simulink library "model_lib"  (Simulink 6.3)
undefined symbols (not defined in the file or in its folder): ADQUANT, alt_alp, alt_delt, alt_gamma, alt_ht, alt_R, alt_T0, atmos, att_trim_IC, constants, dc_L2W_IC, DiscIntNeverNeededParam, dtsim, enforce_fuel, inertia_maxprop, inertia_noprop, latlonh_IC, MACH, MACH_att_int_IC, MACH_att_Kb, MACH_att_Kc, MACH_att_Ki, MACH_pos_IC, MACH_pos_int_IC, MACH_pos_Kb, MACH_pos_Kc, MACH_pos_Ki, MACH_pqr_IC, MACH_pqr_int_IC, MACH_pqr_Kb, MACH_pqr_Kc, MACH_pqr_Ki, MACH_quat_IC, MACH_vel_IC, MACH_vel_int_IC, MACH_vel_Kb, MACH_vel_Kc, MACH_vel_Ki, mass_maxprop, mass_noprop, obac_params, r_accel, r_cg_maxprop, r_cg_noprop, r_prop, rho_sl, SENS, SERVO, throttle_idx, tvc_idx, use_NdEdh_pos, use_wind_meas_sim, use_xdot_ground, vehicle_params
libraries: utility_lib x22, model_lib x18, simulink x14, aerospace x1
(part 1 of 2)
settings Model: LastModifiedBy=E700252  ExtModeAutoUpdateStatusClock=off  StrictBusMsg=None

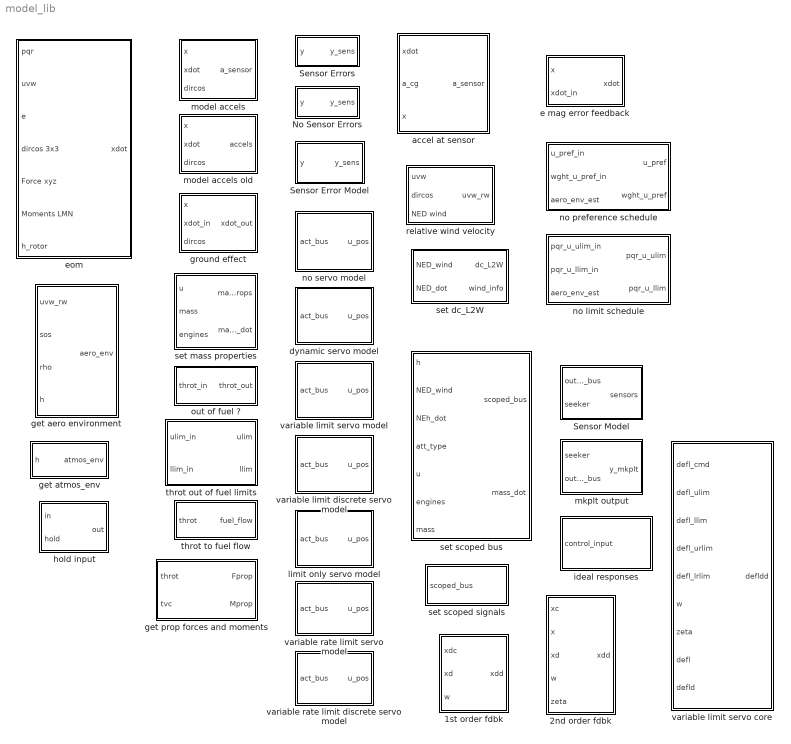
== system model_lib ==
  1st order fdbk : Subsystem
  2nd order fdbk : Subsystem
  No Sensor Errors : Subsystem
  Sensor Error Model : Subsystem  BlockChoice=No Sensor Errors
      settings: TemplateBlock=self  MemberBlocks=No Sensor Errors,Sensor Errors
  Sensor Errors : Subsystem
  Sensor Model : Subsystem
  accel at sensor : Subsystem  mask{vehicle_params=vehicle_params}
      mask prompts: vehicle_params "vehicle params"
      mask init:
      | paramnames = fieldnames(vehicle_params);
      | for i=1:length(paramnames)
      | 	eval([paramnames{i} '= vehicle_params.' paramnames{i} ';']);
      | end
  dynamic servo model : Subsystem
  e mag error feedback : Subsystem
  eom : Subsystem
  get aero environment : Subsystem
  get atmos_env : Subsystem  mask{atmos_params=atmos}
      mask prompts: atmos_params "atmos params"
      mask init:
      | paramnames = fieldnames(atmos_params);
      | for i=1:length(paramnames)
      | 	eval([paramnames{i} '= atmos_params.' paramnames{i} ';']);
      | end
  get prop forces and moments : Subsystem
  ground effect : Subsystem  mask{vehicle_params=vehicle_params}
      mask prompts: vehicle_params "vehicle params"
      mask init:
      | num_x = vehicle_params.num_x;
  hold input : Subsystem
  ideal responses : Subsystem
  limit only servo model : Subsystem
  mkplt output : Subsystem
  model accels : Subsystem  mask{vehicle_params=vehicle_params}
      mask prompts: vehicle_params "vehicle params"
      mask init:
      | paramnames = fieldnames(vehicle_params);
      | for i=1:length(paramnames)
      | 	eval([paramnames{i} '= vehicle_params.' paramnames{i} ';']);
      | end
  model accels old : Subsystem  mask{vehicle_params=vehicle_params}
      mask prompts: vehicle_params "vehicle params"
      mask init:
      | lxa = vehicle_params.lxa;
      | lya = vehicle_params.lya;
      | lza = vehicle_params.lza;
      | num_x = vehicle_params.num_x;
      | 
      | if isfield(vehicle_params,'zero_pqr_dot')
      | 	zero_pqr_dot = vehicle_params.zero_pqr_dot;
      | else
      | 	zero_pqr_dot = 0;
      | end
  no limit schedule : Subsystem
  no preference schedule : Subsystem
  no servo model : Subsystem
  out of fuel ? : Subsystem
  relative wind velocity : Subsystem
  set dc_L2W : Subsystem
  set mass properties : Subsystem  mask{vehicle_params=vehicle_params}
      mask prompts: vehicle_params "vehicle params"
      mask init:
      | paramnames = fieldnames(vehicle_params);
      | for i=1:length(paramnames)
      | 	eval([paramnames{i} '= vehicle_params.' paramnames{i} ';']);
      | end
  set scoped bus : Subsystem  mask{vehicle_params=obac_params}
      mask prompts: vehicle_params "vehicle params"
  set scoped signals : Subsystem
  throt out of fuel limits : Subsystem
  throt to fuel flow : Subsystem
  variable limit discrete servo model : Subsystem
  variable limit servo core : Subsystem
  variable limit servo model : Subsystem
  variable rate limit discrete servo model : Subsystem
  variable rate limit servo model : Subsystem

== system model_lib/1st order fdbk ==
  xdc : Inport
  xd : Inport  Port=2
  w : Inport  Port=3
  Product1 : Product  RndMeth=Zero
  Sum1 : Sum  Inputs=|+-
  xdd : Outport
  wires:
  Product1/1 -> xdd/1
  w/1 -> Product1/2
  xd/1 -> Sum1/2
  xdc/1 -> Sum1/1
  Sum1/1 -> Product1/1

== system model_lib/2nd order fdbk ==
  xc : Inport
  x : Inport  Port=2
  xd : Inport  Port=3
  w : Inport  Port=4
  zeta : Inport  Port=5
  Gain : Gain  Gain=2
  Product1 : Product  Inputs=3  RndMeth=Zero
  Product2 : Product  Inputs=3  RndMeth=Zero
  Sum1 : Sum  Inputs=|+-
  Sum2 : Sum  Inputs=|+-
  xdd : Outport
  wires:
  Gain/1 -> Product2/2
  xd/1 -> Product2/3
  zeta/1 -> Gain/1
  Product2/1 -> Sum2/2
  Sum2/1 -> xdd/1
  Product1/1 -> Sum2/1
  w/1 -> Product2/1, Product1/3, Product1/2
  x/1 -> Sum1/2
  xc/1 -> Sum1/1
  Sum1/1 -> Product1/1

== system model_lib/No Sensor Errors ==
  note: Sensors
  y : Inport
  y_sens : Outport
  wires:
  y/1 -> y_sens/1

== system model_lib/Sensor Error Model ==
  y : Inport
  No Sensor Errors : model_lib/No Sensor Errors
  y_sens : Outport
  wires:
  y/1 -> No Sensor Errors/1
  No Sensor Errors/1 -> y_sens/1

== system model_lib/Sensor Errors ==
  note: Sensors
  y : Inport
  Sensor A/D Quantization : Subsystem
  Sensor Errors : Subsystem
  y_sens : Outport
  wires:
  Sensor Errors/1(ys) -> Sensor A/D Quantization/1(y)
  Sensor A/D Quantization/1(yQ) -> y_sens/1
  y/1 -> Sensor Errors/1(y)

== system model_lib/Sensor Model ==
  note: Note: dircos is the DCM
      | for the quaternion state
  output_bus : Inport
  seeker : Inport  Port=2
  Bus Creator : BusCreator  Inputs=9
  Bus Selector : BusSelector  OutputSignals=x,xdot,y.accels_cg,y.dircos,u_servo,NED_wind
  Constant : Constant
  Gain1 : Gain  Gain=[1 1 -1]  SaturateOnIntegerOverflow=on
  NEh : Selector  Elements=MACH.NEh_idx  InputPortWidth=MACH.num_x
  NEh2LLh : utility_lib/NEh2LLh
  NEh_dot : Selector  Elements=MACH.NEh_idx  InputPortWidth=MACH.num_x
  Signal Specification : SignalSpecification
  Terminator : Terminator
  initial position : Constant  Value=latlonh_IC
  pqr : Selector  Elements=MACH.pqr_idx  InputPortWidth=MACH.num_x
  quat : Selector  Elements=MACH.quat_idx  InputPortWidth=MACH.num_x
  use_wind_meas_sim : Gain  Gain=use_wind_meas_sim  SaturateOnIntegerOverflow=on
  sensors : Outport
  wires:
  Bus Selector/4 -> Terminator/1  "<dircos>"
  Bus Selector/3 -> Bus Creator/5  "<accels_cg>"
  Bus Selector/1 -> pqr/1, NEh/1, quat/1  "<x>"
  seeker/1 -> Bus Creator/9  "seeker"
  Bus Selector/6 -> use_wind_meas_sim/1  "<NED_wind>"
  output_bus/1 -> Bus Selector/1
  NEh/1 -> NEh2LLh/1
  Constant/1 -> Bus Creator/6  "nav_ok"
  initial position/1 -> NEh2LLh/2
  quat/1 -> Bus Creator/3  "e"
  Bus Selector/2 -> NEh_dot/1  "<xdot>"
  NEh_dot/1 -> Gain1/1  "NEh_dot"
  Bus Creator/1 -> sensors/1
  pqr/1 -> Bus Creator/1  "pqr"
  NEh2LLh/1 -> Bus Creator/2  "latlonh"
  Gain1/1 -> Bus Creator/4  "NED_dot"
  use_wind_meas_sim/1 -> Bus Creator/8  "NED_wind"
  Bus Selector/5 -> Signal Specification/1  "<u_servo>"
  Signal Specification/1 -> Bus Creator/7  "u_meas"

== system model_lib/accel at sensor ==
  xdot : Inport
  a_cg : Inport  Port=2
  x : Inport  Port=3
  Product : Product  RndMeth=Zero
  Product1 : Product  RndMeth=Zero
  Sum : Sum  Inputs=+-|
  Sum1 : Sum  Inputs=|+-  SaturateOnIntegerOverflow=on  InputSameDT=on
  Sum10 : Sum  Inputs=+++  SaturateOnIntegerOverflow=on  InputSameDT=on
  accel location : Constant  Value=r_accel
  pqr : Selector  Elements=pqr_idx  InputPortWidth=num_x
  pqr . l_sensor : simulink/Math Operations/Dot Product  InputSameDT=on  OutDataType=sfix(16)  OutScaling=2^-10  DoSatur=off
  pqr . pqr : simulink/Math Operations/Dot Product  InputSameDT=on  OutDataType=sfix(16)  OutScaling=2^-10  DoSatur=off
  pqr_dot : Selector  Elements=pqr_idx  InputPortWidth=num_x
  pqr_dot x l_sensor : utility_lib/cross product
  a_sensor : Outport
  wires:
  Sum1/1 -> Sum10/3
  pqr_dot x l_sensor/1 -> Sum10/2
  a_cg/1 -> Sum10/1
  Product1/1 -> Sum1/2
  Product/1 -> Sum1/1
  pqr . pqr/1 -> Product1/2
  pqr . l_sensor/1 -> Product/1
  x/1 -> pqr/1
  xdot/1 -> pqr_dot/1
  Sum10/1 -> a_sensor/1
  accel location/1 -> Sum/1
  [r_cg] -> Sum/2
  Sum/1 -> Product1/1, pqr . l_sensor/1, pqr_dot x l_sensor/2  "l_sensor"
  pqr_dot/1 -> pqr_dot x l_sensor/1
  pqr/1 -> Product/2, pqr . pqr/2, pqr . pqr/1, pqr . l_sensor/2

== system model_lib/dynamic servo model ==
  note: DYNAMIC SERVO MODEL
      | W^2*e^(-sT) / (S^2 + 2*Z*Ws + W^2)
  act_bus : Inport
  2*Z*W : Gain  Orientation=left  Gain=2*SERVO.z.*SERVO.w  SaturateOnIntegerOverflow=on
  Bus Selector : BusSelector  OutputSignals=u_cmd
  Sum : Sum  Inputs=|+-  SaturateOnIntegerOverflow=on  InputSameDT=on
  Sum1 : Sum  Inputs=|+-  SaturateOnIntegerOverflow=on  InputSameDT=on
  Transport Delay : TransportDelay  DelayTime=SERVO.delay  InitialOutput=SERVO.x0  PadeOrder=2
  W^2 : Gain  Gain=SERVO.w.^2  SaturateOnIntegerOverflow=on
  pos integrator : Integrator  InitialCondition=SERVO.x0  LimitOutput=on  UpperSaturationLimit=SERVO.ulim  LowerSaturationLimit=SERVO.llim
  rate integrator : Integrator  LimitOutput=on  UpperSaturationLimit=SERVO.urlim  LowerSaturationLimit=SERVO.lrlim
  u_pos : Outport
  wires:
  Sum/1 -> W^2/1
  W^2/1 -> Sum1/1
  2*Z*W/1 -> Sum1/2
  rate integrator/1 -> 2*Z*W/1, pos integrator/1
  pos integrator/1 -> Sum/2, u_pos/1
  Sum1/1 -> rate integrator/1
  act_bus/1 -> Bus Selector/1
  Transport Delay/1 -> Sum/1
  Bus Selector/1 -> Transport Delay/1  "<u_cmd>"

== system model_lib/e mag error feedback ==
  x : Inport
  xdot_in : Inport  Port=2
  Assignment : Assignment  Elements=MACH.quat_idx  OutputInitialize=Initialize using input (U1)
  Constant : Constant  Orientation=up
  Constant2 : Constant  Value=0.001
  Gain : Gain  Gain=MACH.K_quaterr/2  SaturateOnIntegerOverflow=on
  Math Function1 : Math  Operator=reciprocal  SaturateOnIntegerOverflow=on
  Math Function2 : Math  Operator=square  SaturateOnIntegerOverflow=on
  MinMax : MinMax  Function=max  Inputs=2
  Product2 : Product  Inputs=**  SaturateOnIntegerOverflow=on  InputSameDT=on
  Sum1 : Sum  Inputs=|-+  SaturateOnIntegerOverflow=on  InputSameDT=on
  Sum2 : Sum  Inputs=+  SaturateOnIntegerOverflow=on  InputSameDT=on
  Sum3 : Sum  Inputs=|++  SaturateOnIntegerOverflow=on  InputSameDT=on
  quat : Selector  Elements=MACH.quat_idx  InputPortWidth=MACH.num_x
  quatdot : Selector  Elements=MACH.quat_idx  InputPortWidth=MACH.num_x
  xdot : Outport
  wires:
  Gain/1 -> Product2/2
  Sum1/1 -> Gain/1
  Constant/1 -> Sum1/2
  Math Function1/1 -> Sum1/1
  Math Function2/1 -> Sum2/1
  Constant2/1 -> MinMax/2
  Sum2/1 -> MinMax/1
  MinMax/1 -> Math Function1/1
  x/1 -> quat/1
  xdot_in/1 -> quatdot/1, Assignment/1
  quat/1 -> Product2/1, Math Function2/1
  Sum3/1 -> Assignment/2
  quatdot/1 -> Sum3/1
  Product2/1 -> Sum3/2
  Assignment/1 -> xdot/1

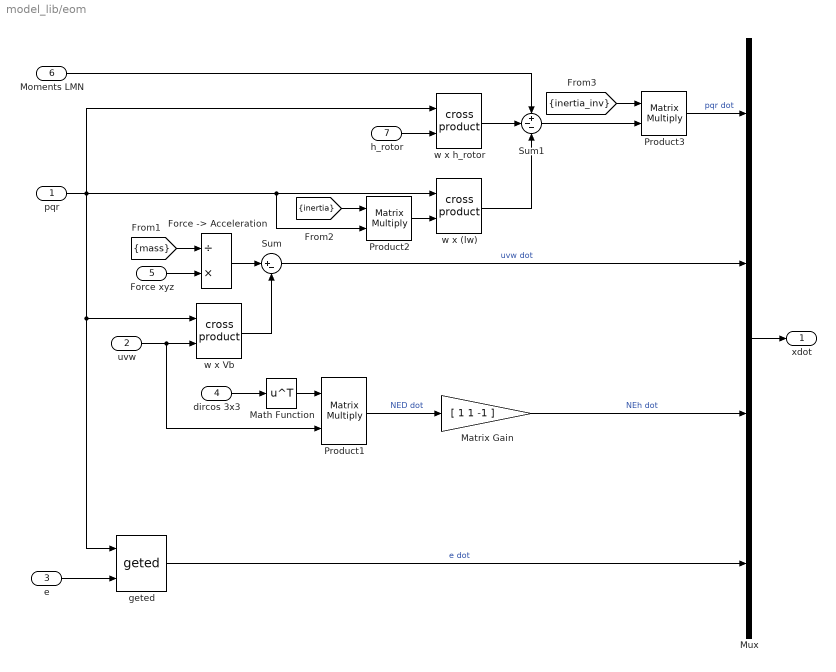
== system model_lib/eom ==
  pqr : Inport
  uvw : Inport  Port=2
  e : Inport  Port=3
  dircos 3x3 : Inport  Port=4
  "Force xyz " : Inport  Port=5
  Moments LMN : Inport  Port=6
  h_rotor : Inport  Port=7
  "Force -> Acceleration" : Product  Inputs=/*  RndMeth=Zero
  Math Function : Math  Operator=transpose  SaturateOnIntegerOverflow=on
  Matrix Gain : Gain  Gain=[ 1 1 -1 ]  SaturateOnIntegerOverflow=on
  Mux : Mux
  Product1 : Product  Multiplication=Matrix(*)  SaturateOnIntegerOverflow=on  InputSameDT=on
  Product2 : Product  Multiplication=Matrix(*)  RndMeth=Zero
  Product3 : Product  Multiplication=Matrix(*)  RndMeth=Zero
  Sum : Sum  Inputs=|+-  SaturateOnIntegerOverflow=on
  Sum1 : Sum  Inputs=+--  SaturateOnIntegerOverflow=on
  geted : utility_lib/geted
  w x (lw) : utility_lib/cross product
  w x Vb : utility_lib/cross product
  w x h_rotor : utility_lib/cross product
  xdot : Outport
  wires:
  Mux/1 -> xdot/1
  geted/1 -> Mux/4  "e dot"
  e/1 -> geted/2
  uvw/1 -> Product1/2, w x Vb/2
  w x Vb/1 -> Sum/2
  "Force xyz "/1 -> "Force -> Acceleration"/2
  Sum/1 -> Mux/2  "uvw dot"
  Matrix Gain/1 -> Mux/3  "NEh dot"
  dircos 3x3/1 -> Math Function/1
  pqr/1 -> geted/1, w x Vb/1, Product2/2, w x (lw)/1, w x h_rotor/1
  Product3/1 -> Mux/1  "pqr dot"
  Product2/1 -> w x (lw)/2
  Moments LMN/1 -> Sum1/1
  Sum1/1 -> Product3/2
  Product1/1 -> Matrix Gain/1  "NED dot"
  Math Function/1 -> Product1/1
  "Force -> Acceleration"/1 -> Sum/1
  h_rotor/1 -> w x h_rotor/2
  w x (lw)/1 -> Sum1/3
  w x h_rotor/1 -> Sum1/2
  [inertia] -> Product2/1
  [mass] -> "Force -> Acceleration"/1
  [inertia_inv] -> Product3/1

== system model_lib/get aero environment ==
  uvw_rw : Inport
  sos : Inport  Port=2  PortDimensions=1
  rho : Inport  Port=3  PortDimensions=1
  h : Inport  Port=4  PortDimensions=1
  Bus Creator : BusCreator  Inputs=9
  Constant : Constant  Value=0.0001
  MinMax : MinMax  Function=max  Inputs=2
  Product1 : Product  RndMeth=Zero
  Product2 : Product  Inputs=*/  RndMeth=Zero
  Signal Specification : SignalSpecification  Dimensions=1
  uvw_rw2Vab : utility_lib/uvw_rw2Vab
  wind_qbar : Fcn  Expr=0.5*u^2
  aero_env : Outport
  wires:
  uvw_rw/1 -> Bus Creator/9, uvw_rw2Vab/1  "uvw_rw"
  uvw_rw2Vab/1 -> MinMax/2
  h/1 -> Bus Creator/8  "h"
  Constant/1 -> MinMax/1
  MinMax/1 -> wind_qbar/1, Product2/1, Signal Specification/1
  Product1/1 -> Bus Creator/4  "qbar"
  rho/1 -> Product1/1, Bus Creator/3  "rho"
  wind_qbar/1 -> Product1/2
  uvw_rw2Vab/3 -> Bus Creator/7  "beta"
  sos/1 -> Product2/2, Bus Creator/2  "sos"
  Product2/1 -> Bus Creator/1  "Mach"
  Bus Creator/1 -> aero_env/1
  Signal Specification/1 -> Bus Creator/5  "vel"
  uvw_rw2Vab/2 -> Bus Creator/6  "alpha"

== system model_lib/get atmos_env ==
  h : Inport
  Bus Creator : BusCreator  Inputs=5
  Gain : Gain  Gain=alt_R*constants.g
  Gain1 : Gain  Gain=alt_gamma*alt_R*constants.g
  Math Function : Math  Operator=sqrt  SaturateOnIntegerOverflow=on
  Product : Product  RndMeth=Zero
  air density : Subsystem
  air temp : Subsystem
  atmos_env : Outport
  wires:
  h/1 -> air temp/1(h), Bus Creator/5, air density/1(h)  "h"
  air temp/1(T) -> Gain1/1, Bus Creator/3, Product/2  "T"
  Gain1/1 -> Math Function/1
  Math Function/1 -> Bus Creator/4  "sos"
  Bus Creator/1 -> atmos_env/1
  air density/1(rho) -> Bus Creator/1, Product/1  "rho"
  Product/1 -> Gain/1
  Gain/1 -> Bus Creator/2  "P"

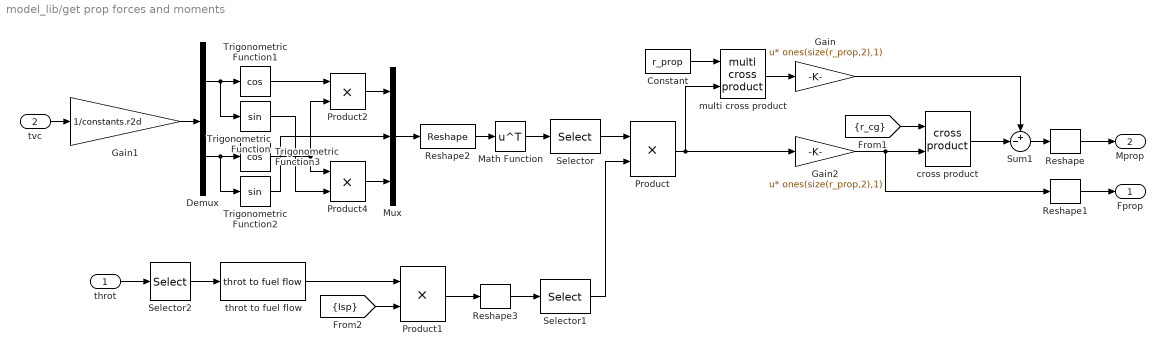
== system model_lib/get prop forces and moments ==
  throt : Inport
  tvc : Inport  Port=2
  Constant : Constant  Value=r_prop  VectorParams1D=off
  Demux : Demux  Outputs=2
  Gain : Gain  Gain=ones(size(r_prop,2),1)  Multiplication=Matrix(u*K)
  Gain1 : Gain  Gain=1/constants.r2d
  Gain2 : Gain  Gain=ones(size(r_prop,2),1)  Multiplication=Matrix(u*K)
  Math Function : Math  Operator=transpose  SaturateOnIntegerOverflow=on
  Mux : Mux  Inputs=3
  Product{,1..2,4} (4 alike) : Product  RndMeth=Zero
  Reshape : simulink/Math Operations/Reshape  OutputDimensionality=1-D array  OutputDimensions=[1,1]
  Reshape1 : simulink/Math Operations/Reshape  OutputDimensionality=1-D array  OutputDimensions=[1,1]
  Reshape2 : simulink/Math Operations/Reshape  OutputDimensionality=Customize  OutputDimensions=[length(tvc_idx)/2 3]
  Reshape3 : simulink/Math Operations/Reshape  OutputDimensionality=Row vector  OutputDimensions=[1,1]
  Selector : Selector  InputType=Matrix  Elements=[1 3]  Rows=-1  Columns=tvc_select  InputPortWidth=3
  Selector1 : Selector  InputType=Matrix  Elements=[1 3]  Rows=ones(1,size(r_prop,2))  Columns=-1  InputPortWidth=3
  Selector2 : Selector  Elements=throt_select  InputPortWidth=length(throttle_idx)
  Sum1 : Sum  Inputs=+-|
  Trigonometric Function : Trigonometry
  Trigonometric Function1 : Trigonometry  Operator=cos
  Trigonometric Function2 : Trigonometry
  Trigonometric Function3 : Trigonometry  Operator=cos
  cross product : utility_lib/cross product
  multi cross product : utility_lib/multi cross product
  throt to fuel flow : model_lib/throt to fuel flow
  Fprop : Outport
  Mprop : Outport  Port=2
  wires:
  Reshape3/1 -> Selector1/1
  Selector1/1 -> Product/2
  Selector/1 -> Product/1
  Math Function/1 -> Selector/1
  Reshape2/1 -> Math Function/1
  Reshape1/1 -> Fprop/1
  Reshape/1 -> Mprop/1
  Sum1/1 -> Reshape/1
  cross product/1 -> Sum1/2
  Gain/1 -> Sum1/1
  multi cross product/1 -> Gain/1
  Gain2/1 -> cross product/2, Reshape1/1
  [r_cg] -> cross product/1
  Product/1 -> multi cross product/2, Gain2/1
  Constant/1 -> multi cross product/1
  tvc/1 -> Gain1/1
  Demux/1 -> Trigonometric Function1/1, Trigonometric Function/1
  Demux/2 -> Trigonometric Function3/1, Trigonometric Function2/1
  Product4/1 -> Mux/3
  Trigonometric Function3/1 -> Product2/2, Product4/1
  throt/1 -> Selector2/1
  Gain1/1 -> Demux/1
  Product2/1 -> Mux/1
  Trigonometric Function1/1 -> Product2/1
  Trigonometric Function/1 -> Product4/2
  Trigonometric Function2/1 -> Mux/2
  [Isp] -> Product1/2
  throt to fuel flow/1 -> Product1/1
  Mux/1 -> Reshape2/1
  Product1/1 -> Reshape3/1
  Selector2/1 -> throt to fuel flow/1

== system model_lib/ground effect ==
  x : Inport
  xdot_in : Inport  Port=2
  dircos : Inport  Port=3
  Matrix Gain1 : Gain  Gain=use_xdot_ground  SaturateOnIntegerOverflow=on
  Selector2 : Selector  Elements=MACH.NEh_idx(3)  InputPortWidth=num_x
  above ground ? : Switch  Criteria=u2 > Threshold  SaturateOnIntegerOverflow=on
  include ground effect : Subsystem
  xdot_out : Outport
  wires:
  xdot_in/1 -> include ground effect/1(xdot_in), above ground ?/1
  dircos/1 -> include ground effect/3(dircos)
  above ground ?/1 -> xdot_out/1
  Selector2/1 -> above ground ?/2  "h"
  x/1 -> include ground effect/2(x), Selector2/1
  Matrix Gain1/1 -> above ground ?/3
  include ground effect/1(xdot_out) -> Matrix Gain1/1

== system model_lib/hold input ==
  in : Inport
  hold : Inport  Port=2
  Constant : Constant
  Memory : Memory  InheritSampleTime=on
  Memory1 : Memory  Orientation=left  InheritSampleTime=on
  Product : Product  RndMeth=Zero
  Switch : Switch  Criteria=u2 ~= 0
  out : Outport
  wires:
  hold/1 -> Product/1
  in/1 -> Switch/3
  Constant/1 -> Memory/1
  Memory/1 -> Product/2
  Product/1 -> Switch/2
  Switch/1 -> out/1, Memory1/1
  Memory1/1 -> Switch/1

== system model_lib/ideal responses ==
  control_input : Inport
      settings: BusObject=control_input_bus
  ideal att rate response : Subsystem
  ideal pos vel response : Subsystem
  wires:
  control_input/1 -> ideal pos vel response/1(control_input), ideal att rate response/1(control_input)

== system model_lib/limit only servo model ==
  note: LIMIT ONLY SERVO MODEL
  act_bus : Inport
  Bus Selector1 : BusSelector  OutputSignals=effector_limits.u_ulim,effector_limits.u_llim,u_cmd
  Enforce lower limit : MinMax  Function=max  Inputs=2  OutScaling=2^-10  ZeroCross=off
  Enforce upper limit : MinMax  Inputs=2  OutScaling=2^-10  ZeroCross=off
  Rate Limiter : RateLimiter  RisingSlewLimit=SERVO.urlim  FallingSlewLimit=SERVO.lrlim  SampleTimeMode=inherited  InitialCondition=SERVO.x0
  u_pos : Outport
  wires:
  Rate Limiter/1 -> u_pos/1
  Enforce lower limit/1 -> Enforce upper limit/2
  Bus Selector1/1 -> Enforce upper limit/1  "<u_ulim>"
  Enforce upper limit/1 -> Rate Limiter/1
  act_bus/1 -> Bus Selector1/1
  Bus Selector1/3 -> Enforce lower limit/2  "<u_cmd>"
  Bus Selector1/2 -> Enforce lower limit/1  "<u_llim>"

== system model_lib/mkplt output ==
  seeker : Inport
  output_bus : Inport  Port=2
  Bus Creator1 : BusCreator  Inputs=10
  Bus Selector : BusSelector  OutputSignals=y.dircos,x,NED_wind
  Bus Selector1 : BusSelector  OutputSignals=mass_props.mass,atmos_env.P,atmos_env.T,dc_L2W
  Gain : Gain  SaturateOnIntegerOverflow=on
  angles : Subsystem
  order outputs as expected by mkplt : BusSelector  OutputSignals=output_bus.y.accels,output_bus.y.accels_cg,output_bus.y.dircos,uvw_rw,tilta;tiltb;cam,phi;theta;psi,mu;alpha;beta,mass,output_bus.y.aero_env,P,T,seeker  OutputAsBus=on
  uvw : Selector  Elements=MACH.uvw_idx  InputPortWidth=MACH.num_x
  y_mkplt : Outport
  wires:
  Bus Selector1/4 -> Bus Creator1/10  "<dc_L2W>"
  Bus Selector1/3 -> Bus Creator1/9  "<T>"
  Bus Selector1/2 -> Bus Creator1/8  "<P>"
  Bus Selector1/1 -> Bus Creator1/7  "<mass>"
  seeker/1 -> Bus Creator1/6  "seeker"
  [scoped_bus] -> Bus Selector1/1
  Bus Selector/2 -> uvw/1  "<x>"
  Bus Creator1/1 -> order outputs as expected by mkplt/1
  Bus Selector/3 -> angles/3(NED_wind)  "<NED_wind>"
  uvw/1 -> angles/2(uvw)
  Bus Selector/1 -> angles/1(dircos)  "<dircos>"
  Gain/1 -> y_mkplt/1
  order outputs as expected by mkplt/1 -> Gain/1
  output_bus/1 -> Bus Creator1/1, Bus Selector/1  "output_bus"
  angles/3(phi;theta;psi) -> Bus Creator1/4  "phi;theta;psi"
  angles/2(tilta;tiltb;cam) -> Bus Creator1/3  "tilta;tiltb;cam"
  angles/1(uvw_rw) -> Bus Creator1/2  "uvw_rw"
  angles/4(mu;alpha;beta) -> Bus Creator1/5  "mu;alpha;beta"

== system model_lib/model accels ==
  x : Inport
  xdot : Inport  Port=2
  dircos : Inport  Port=3
  Gain2 : Gain  Gain=constants.g  SaturateOnIntegerOverflow=on
  accel at cg : Subsystem
  accel at sensor : model_lib/accel at sensor  vehicle_params=vehicle_params
  dircos(:,3) : Selector  Elements=7:9  InputPortWidth=9
  pqr : Selector  Elements=pqr_idx  InputPortWidth=num_x
  uvw : Selector  Elements=uvw_idx  InputPortWidth=num_x
  uvw_dot : Selector  Elements=uvw_idx  InputPortWidth=num_x
  a_sensor : Outport
  wires:
  x/1 -> uvw/1, pqr/1, accel at sensor/3
  dircos(:,3)/1 -> Gain2/1
  xdot/1 -> uvw_dot/1, accel at sensor/1
  dircos/1 -> dircos(:,3)/1
  uvw_dot/1 -> accel at cg/1(uvw_dot)
  accel at sensor/1 -> a_sensor/1
  accel at cg/1(a_cg) -> accel at sensor/2
  Gain2/1 -> accel at cg/2(gvec)
  uvw/1 -> accel at cg/3(uvw)
  pqr/1 -> accel at cg/4(pqr)

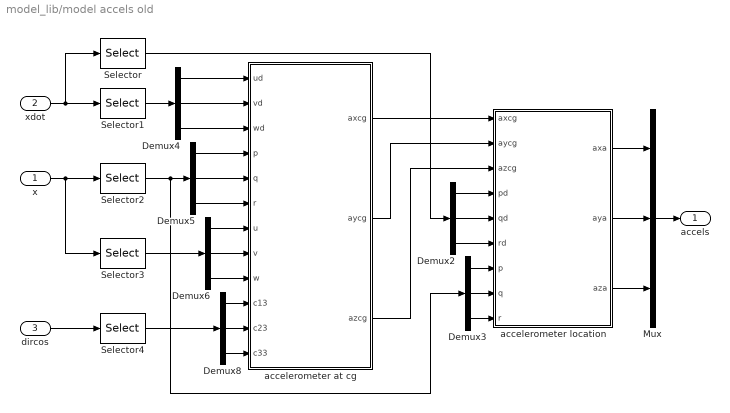
== system model_lib/model accels old ==
  x : Inport
  xdot : Inport  Port=2
  dircos : Inport  Port=3
  Demux{2..6,8} (6 alike) : Demux  Outputs=3
  Mux : Mux  Inputs=[1 1 1]
  Selector : Selector  Elements=MACH.pqr_idx  InputPortWidth=num_x
  Selector1 : Selector  Elements=MACH.uvw_idx  InputPortWidth=num_x
  Selector2 : Selector  Elements=MACH.pqr_idx  InputPortWidth=num_x
  Selector3 : Selector  Elements=MACH.uvw_idx  InputPortWidth=num_x
  Selector4 : Selector  Elements=7:9  InputPortWidth=9
  accelerometer at cg : Subsystem
  accelerometer location : Subsystem
  accels : Outport
  wires:
  accelerometer at cg/1(axcg) -> accelerometer location/1(axcg)
  accelerometer at cg/2(aycg) -> accelerometer location/2(aycg)
  accelerometer at cg/3(azcg) -> accelerometer location/3(azcg)
  Mux/1 -> accels/1
  accelerometer location/1(axa) -> Mux/1
  accelerometer location/2(aya) -> Mux/2
  accelerometer location/3(aza) -> Mux/3
  Demux2/1 -> accelerometer location/4(pd)
  Demux2/2 -> accelerometer location/5(qd)
  Demux2/3 -> accelerometer location/6(rd)
  Demux3/1 -> accelerometer location/7(p)
  Demux3/2 -> accelerometer location/8(q)
  Demux3/3 -> accelerometer location/9(r)
  Demux4/1 -> accelerometer at cg/1(ud)
  Demux4/2 -> accelerometer at cg/2(vd)
  Demux5/1 -> accelerometer at cg/4(p)
  Demux5/2 -> accelerometer at cg/5(q)
  Demux5/3 -> accelerometer at cg/6(r)
  Demux6/1 -> accelerometer at cg/7(u)
  Demux6/2 -> accelerometer at cg/8(v)
  Demux6/3 -> accelerometer at cg/9(w)
  Demux4/3 -> accelerometer at cg/3(wd)
  Selector1/1 -> Demux4/1
  Selector2/1 -> Demux5/1, Demux3/1
  Selector3/1 -> Demux6/1
  dircos/1 -> Selector4/1
  Demux8/1 -> accelerometer at cg/10(c13)
  Demux8/2 -> accelerometer at cg/11(c23)
  Demux8/3 -> accelerometer at cg/12(c33)
  xdot/1 -> Selector1/1, Selector/1
  Selector4/1 -> Demux8/1
  x/1 -> Selector2/1, Selector3/1
  Selector/1 -> Demux2/1

== system model_lib/no limit schedule ==
  note: NO LIMIT SCHEDULE
  pqr_u_ulim_in : Inport
  pqr_u_llim_in : Inport  Port=2
  aero_env_est : Inport  Port=3
  Terminator : Terminator
  pqr_u_ulim : Outport
  pqr_u_llim : Outport  Port=2
  wires:
  pqr_u_llim_in/1 -> pqr_u_llim/1
  pqr_u_ulim_in/1 -> pqr_u_ulim/1
  aero_env_est/1 -> Terminator/1

== system model_lib/no preference schedule ==
  note: NO PREFERENCE SCHEDULE
  u_pref_in : Inport
  wght_u_pref_in : Inport  Port=2
  aero_env_est : Inport  Port=3
  Terminator : Terminator
  u_pref : Outport
  wght_u_pref : Outport  Port=2
  wires:
  u_pref_in/1 -> u_pref/1
  wght_u_pref_in/1 -> wght_u_pref/1
  aero_env_est/1 -> Terminator/1

== system model_lib/no servo model ==
  note: NO SERVO MODEL
  act_bus : Inport
  Bus Selector : BusSelector  OutputSignals=u_cmd
  u_pos : Outport
  wires:
  act_bus/1 -> Bus Selector/1
  Bus Selector/1 -> u_pos/1  "<u_cmd>"

== system model_lib/out of fuel ? ==
  throt_in : Inport
  Compare To Zero : simulink/Logic and Bit Operations/Compare To Zero  relop=<=  LogicOutDataTypeMode=boolean  ZeroCross=off
  Constant : Constant  Value=enforce_fuel
  Logical Operator : Logic  Operator=NAND  AllPortsSameDT=off  OutDataTypeMode=Boolean
  Product : Product  RndMeth=Zero
  throt_out : Outport
  wires:
  Product/1 -> throt_out/1
  [fuel] -> Compare To Zero/1
  throt_in/1 -> Product/1
  Compare To Zero/1 -> Logical Operator/1
  Constant/1 -> Logical Operator/2
  Logical Operator/1 -> Product/2

== system model_lib/relative wind velocity ==
  uvw : Inport
  dircos : Inport  Port=2
  NED wind : Inport  Port=3
  Product : Product  Multiplication=Matrix(*)  SaturateOnIntegerOverflow=on
  Reshape : simulink/Math Operations/Reshape  OutputDimensionality=Customize  OutputDimensions=[3,3]
  Sum1 : Sum  Inputs=++|  SaturateOnIntegerOverflow=on
  uvw_rw : Outport
  wires:
  dircos/1 -> Reshape/1
  uvw/1 -> Sum1/2
  NED wind/1 -> Product/2
  Product/1 -> Sum1/1
  Sum1/1 -> uvw_rw/1
  Reshape/1 -> Product/1

== system model_lib/set dc_L2W ==
  NED_wind : Inport
  NED_dot : Inport  Port=2
  Bus Creator : BusCreator  Inputs=3
  Bus Selector : BusSelector  OutputSignals=Rslant,azimuth,elevation
  Signal Specification : SignalSpecification
  Signal Specification1 : SignalSpecification
  Signal Specification2 : SignalSpecification
  Sum : Sum  Inputs=|++
  vec2dc : utility_lib/vec2dc
  dc_L2W : Outport
  wind_info : Outport  Port=2
  wires:
  Sum/1 -> vec2dc/1
  NED_wind/1 -> Sum/1
  NED_dot/1 -> Sum/2
  vec2dc/1 -> dc_L2W/1
  vec2dc/2 -> Bus Selector/1
  Bus Selector/1 -> Signal Specification/1  "<Rslant>"
  Bus Selector/2 -> Signal Specification1/1  "<azimuth>"
  Bus Selector/3 -> Signal Specification2/1  "<elevation>"
  Bus Creator/1 -> wind_info/1
  Signal Specification/1 -> Bus Creator/1  "vel_rw"
  Signal Specification1/1 -> Bus Creator/2  "chi_rw"
  Signal Specification2/1 -> Bus Creator/3  "gamma_rw"

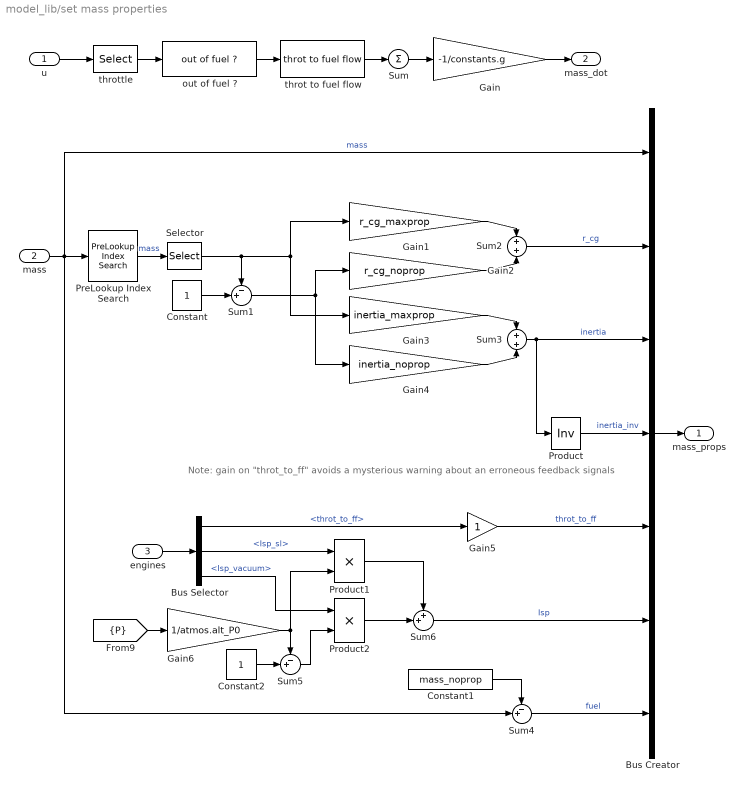
== system model_lib/set mass properties ==
  note: Note: gain on "throt_to_ff" avoids
      |  a mysterious warning about an
      | erroneous feedback signals
  u : Inport
  mass : Inport  Port=2
  engines : Inport  Port=3
  Bus Creator : BusCreator  Inputs=7
  Bus Selector : BusSelector  OutputSignals=throt_to_ff,Isp_sl,Isp_vacuum
  Constant : Constant
  Constant1 : Constant  Value=mass_noprop
  Constant2 : Constant
  Gain : Gain  Gain=-1/constants.g
  Gain1 : Gain  Gain=r_cg_maxprop
  Gain2 : Gain  Gain=r_cg_noprop
  Gain3 : Gain  Gain=inertia_maxprop
  Gain4 : Gain  Gain=inertia_noprop
  Gain5 : Gain
  Gain6 : Gain  Gain=1/atmos.alt_P0
  PreLookup Index Search : simulink/Lookup Tables/PreLookup Index Search  bpData=[mass_noprop max(mass_maxprop,mass_noprop+1)]  searchMode=Binary Search  cacheBpFlag=off  outputFlag=off  IndexDataType=uint32  extrapMode=Clip to Range  rangeErrorMode=None
  Product : Product  Inputs=/  Multiplication=Matrix(*)  RndMeth=Zero
  Product1 : Product  RndMeth=Zero
  Product2 : Product  RndMeth=Zero
  Selector : Selector  Elements=2  InputPortWidth=2
  Sum : Sum  Inputs=+
  Sum1 : Sum  Inputs=-+|
  Sum2 : Sum  Inputs=+|+
  Sum3 : Sum  Inputs=+|+
  Sum4 : Sum  Inputs=-+|
  Sum5 : Sum  Inputs=-+|
  Sum6 : Sum  Inputs=++|
  out of fuel ? : model_lib/out of fuel ?
  throt to fuel flow : model_lib/throt to fuel flow
  throttle : Selector  Elements=MACH.throttle_idx  InputPortWidth=MACH.num_u
  mass_props : Outport
  mass_dot : Outport  Port=2
  wires:
  Gain5/1 -> Bus Creator/5  "throt_to_ff"
  Product2/1 -> Sum6/2
  Product1/1 -> Sum6/1
  Sum5/1 -> Product2/2
  Constant2/1 -> Sum5/2
  Gain6/1 -> Sum5/1, Product1/2
  Bus Selector/3 -> Product2/1  "<Isp_vacuum>"
  [P] -> Gain6/1
  Bus Selector/2 -> Product1/1  "<Isp_sl>"
  engines/1 -> Bus Selector/1
  Product/1 -> Bus Creator/4  "inertia_inv"
  Constant1/1 -> Sum4/1
  Sum4/1 -> Bus Creator/7  "fuel"
  out of fuel ?/1 -> throt to fuel flow/1
  Gain/1 -> mass_dot/1
  Sum3/1 -> Bus Creator/3, Product/1  "inertia"
  Sum2/1 -> Bus Creator/2  "r_cg"
  Gain4/1 -> Sum3/2
  Gain3/1 -> Sum3/1
  Gain2/1 -> Sum2/2
  Gain1/1 -> Sum2/1
  Sum1/1 -> Gain4/1, Gain2/1
  Constant/1 -> Sum1/2
  Selector/1 -> Gain3/1, Gain1/1, Sum1/1
  mass/1 -> Bus Creator/1, Sum4/2, PreLookup Index Search/1  "mass"
  Sum/1 -> Gain/1
  throt to fuel flow/1 -> Sum/1
  Bus Creator/1 -> mass_props/1
  throttle/1 -> out of fuel ?/1
  u/1 -> throttle/1
  Sum6/1 -> Bus Creator/6  "Isp"
  PreLookup Index Search/1 -> Selector/1  "mass"
  Bus Selector/1 -> Gain5/1  "<throt_to_ff>"

== system model_lib/set scoped bus ==
  note: Note: gain on "att_type" avoids
      |  a mysterious warning about an
      | erroneous feedback signals
  h : Inport
  NED_wind : Inport  Port=2
  NEh_dot : Inport  Port=3
  att_type : Inport  Port=4
  u : Inport  Port=5
  engines : Inport  Port=6
  mass : Inport  Port=7
  Bus Creator : BusCreator  Inputs=5
  Gain : Gain  Gain=[1 1 -1]  SaturateOnIntegerOverflow=on
  Gain1 : Gain
  get atmos_env : model_lib/get atmos_env  atmos_params=atmos
  set dc_L2W : model_lib/set dc_L2W
  set mass properties : model_lib/set mass properties  vehicle_params=vehicle_params
  scoped_bus : Outport
  mass_dot : Outport  Port=2
  wires:
  Gain1/1 -> Bus Creator/4  "att_type"
  engines/1 -> set mass properties/3
  Gain/1 -> set dc_L2W/2
  mass/1 -> set mass properties/2
  att_type/1 -> Gain1/1
  NEh_dot/1 -> Gain/1
  h/1 -> get atmos_env/1
  u/1 -> set mass properties/1
  NED_wind/1 -> set dc_L2W/1
  set dc_L2W/1 -> Bus Creator/2  "dc_L2W"
  Bus Creator/1 -> scoped_bus/1
  set mass properties/2 -> mass_dot/1
  set mass properties/1 -> Bus Creator/5  "mass_props"
  get atmos_env/1 -> Bus Creator/1  "atmos_env"
  set dc_L2W/2 -> Bus Creator/3  "wind_info"

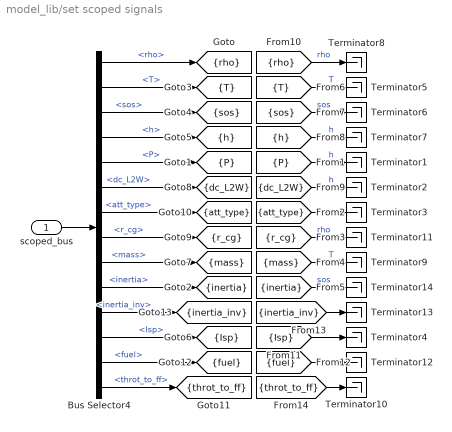
== system model_lib/set scoped signals ==
  scoped_bus : Inport
  Bus Selector4 : BusSelector  OutputSignals=atmos_env.rho,atmos_env.T,atmos_env.sos,atmos_env.h,atmos_env.P,dc_L2W,att_type,mass_props.r_cg,mass_props.mass,mass_props.inertia,mass_props.inertia_inv,mass_props.Isp,mass_props.fuel,mass_props.throt_to_ff
  Terminator{1..14} (14 alike) : Terminator
  tag scope: Isp=scoped, P=scoped, T=scoped, att_type=scoped, dc_L2W=scoped, fuel=scoped, h=scoped, inertia=scoped, inertia_inv=scoped, mass=scoped, r_cg=scoped, rho=scoped, sos=scoped, throt_to_ff=scoped
  wires:
  [throt_to_ff] -> Terminator10/1
  Bus Selector4/14 -> [throt_to_ff]  "<throt_to_ff>"
  Bus Selector4/11 -> [inertia_inv]  "<inertia_inv>"
  [inertia_inv] -> Terminator13/1
  [fuel] -> Terminator12/1
  Bus Selector4/13 -> [fuel]  "<fuel>"
  [Isp] -> Terminator4/1
  [inertia] -> Terminator14/1  "sos"
  [mass] -> Terminator9/1  "T"
  [r_cg] -> Terminator11/1  "rho"
  [att_type] -> Terminator3/1
  [dc_L2W] -> Terminator2/1  "h"
  [P] -> Terminator1/1  "h"
  [rho] -> Terminator8/1  "rho"
  [T] -> Terminator5/1  "T"
  [sos] -> Terminator6/1  "sos"
  [h] -> Terminator7/1  "h"
  Bus Selector4/12 -> [Isp]  "<Isp>"
  Bus Selector4/10 -> [inertia]  "<inertia>"
  Bus Selector4/9 -> [mass]  "<mass>"
  Bus Selector4/8 -> [r_cg]  "<r_cg>"
  Bus Selector4/7 -> [att_type]  "<att_type>"
  Bus Selector4/6 -> [dc_L2W]  "<dc_L2W>"
  Bus Selector4/5 -> [P]  "<P>"
  Bus Selector4/4 -> [h]  "<h>"
  Bus Selector4/3 -> [sos]  "<sos>"
  Bus Selector4/2 -> [T]  "<T>"
  Bus Selector4/1 -> [rho]  "<rho>"
  scoped_bus/1 -> Bus Selector4/1

== system model_lib/throt out of fuel limits ==
  ulim_in : Inport
  llim_in : Inport  Port=2
  Assignment : Assignment  Elements=MACH.throttle_idx  OutputInitialize=Initialize using input (U1)
  Assignment1 : Assignment  Elements=MACH.throttle_idx  OutputInitialize=Initialize using input (U1)
  out of fuel llim : model_lib/out of fuel ?
  out of fuel ulim : model_lib/out of fuel ?
  throttle llim : Selector  Elements=MACH.throttle_idx  InputPortWidth=MACH.num_u
  throttle ulim : Selector  Elements=MACH.throttle_idx  InputPortWidth=MACH.num_u
  ulim : Outport
  llim : Outport  Port=2
  wires:
  ulim_in/1 -> throttle ulim/1, Assignment1/1
  llim_in/1 -> Assignment/1, throttle llim/1
  out of fuel ulim/1 -> Assignment1/2
  throttle ulim/1 -> out of fuel ulim/1
  out of fuel llim/1 -> Assignment/2
  Assignment1/1 -> ulim/1
  Assignment/1 -> llim/1
  throttle llim/1 -> out of fuel llim/1

== system model_lib/throt to fuel flow ==
  throt : Inport
  Product : Product  RndMeth=Zero
  fuel_flow : Outport
  wires:
  throt/1 -> Product/1
  [throt_to_ff] -> Product/2
  Product/1 -> fuel_flow/1

== system model_lib/variable limit discrete servo model ==
  note: VARIABLE LIMIT DISCRETE SERVO MODEL
  act_bus : Inport
  2*Z*W : Gain  Orientation=left  Gain=2*SERVO.z.*SERVO.w  SaturateOnIntegerOverflow=on
  Bus Selector1 : BusSelector  OutputSignals=effector_limits.u_ulim,effector_limits.u_llim,u_cmd
  Enforce lower limit : MinMax  Function=max  Inputs=2  OutScaling=2^-10  ZeroCross=off
  Enforce upper limit : MinMax  Inputs=2  OutScaling=2^-10  ZeroCross=off
  Rate Limiter : RateLimiter  RisingSlewLimit=SERVO.urlim  FallingSlewLimit=SERVO.lrlim  SampleTimeMode=inherited  InitialCondition=SERVO.x0
  Sum : Sum  Inputs=|+-  SaturateOnIntegerOverflow=on  InputSameDT=on
  Sum1 : Sum  Inputs=|++  SaturateOnIntegerOverflow=on  InputSameDT=on
  Sum2 : Sum  Orientation=left  Inputs=-+|  SaturateOnIntegerOverflow=on  InputSameDT=on
  Sum3 : Sum  Inputs=|+-  SaturateOnIntegerOverflow=on  InputSameDT=on
  W^2 : Gain  Gain=SERVO.w.^2  SaturateOnIntegerOverflow=on
  anti-windup gain : Gain  Orientation=left  Gain=SERVO.pos_Kaw
  pos integrator : DiscreteIntegrator  InitialCondition=SERVO.x0  SampleTime=-1  ICPrevOutput=DiscIntNeverNeededParam  ICPrevScaledInput=DiscIntNeverNeededParam
  rate integrator : DiscreteIntegrator  SampleTime=-1  LimitOutput=on  UpperSaturationLimit=SERVO.urlim  LowerSaturationLimit=SERVO.lrlim  ICPrevOutput=DiscIntNeverNeededParam  ICPrevScaledInput=DiscIntNeverNeededParam
  u_pos : Outport
  wires:
  Enforce upper limit/1 -> Rate Limiter/1
  Enforce lower limit/1 -> Enforce upper limit/2
  pos integrator/1 -> Sum2/1, Enforce lower limit/2
  Sum2/1 -> anti-windup gain/1
  anti-windup gain/1 -> Sum1/2
  Sum1/1 -> pos integrator/1
  rate integrator/1 -> Sum1/1, 2*Z*W/1
  Sum/1 -> W^2/1
  Sum3/1 -> rate integrator/1
  W^2/1 -> Sum3/1
  2*Z*W/1 -> Sum3/2
  Rate Limiter/1 -> u_pos/1, Sum2/2, Sum/2
  act_bus/1 -> Bus Selector1/1
  Bus Selector1/3 -> Sum/1  "<u_cmd>"
  Bus Selector1/2 -> Enforce lower limit/1  "<u_llim>"
  Bus Selector1/1 -> Enforce upper limit/1  "<u_ulim>"

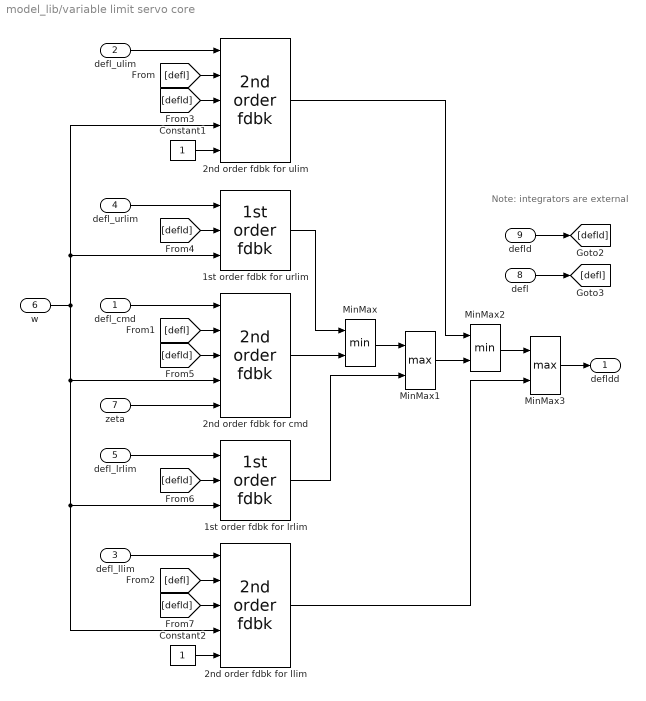
== system model_lib/variable limit servo core ==
  note: Note: integrators are external
  defl_cmd : Inport  OutDataType=fixdt(1,16,0)  OutScaling=[]
  defl_ulim : Inport  Port=2  OutDataType=fixdt(1,16,0)  OutScaling=[]
  defl_llim : Inport  Port=3
  defl_urlim : Inport  Port=4  OutDataType=fixdt(1,16,0)  OutScaling=[]
  defl_lrlim : Inport  Port=5  OutDataType=fixdt(1,16,0)  OutScaling=[]
  w : Inport  Port=6  OutDataType=fixdt(1,16,0)  OutScaling=[]
  zeta : Inport  Port=7  OutDataType=fixdt(1,16,0)  OutScaling=[]
  defl : Inport  Port=8  OutDataType=fixdt(1,16,0)  OutScaling=[]
  defld : Inport  Port=9  OutDataType=fixdt(1,16,0)  OutScaling=[]
  1st order fdbk for lrlim : model_lib/1st order fdbk
  1st order fdbk for urlim : model_lib/1st order fdbk
  2nd order fdbk for cmd : model_lib/2nd order fdbk
  2nd order fdbk for llim : model_lib/2nd order fdbk
  2nd order fdbk for ulim : model_lib/2nd order fdbk
  Constant1 : Constant
  Constant2 : Constant
  MinMax : MinMax  Inputs=2
  MinMax1 : MinMax  Function=max  Inputs=2
  MinMax2 : MinMax  Inputs=2
  MinMax3 : MinMax  Function=max  Inputs=2
  defldd : Outport  OutDataType=fixdt(1,16,0)  OutScaling=[]
  wires:
  MinMax/1 -> MinMax1/1
  defl_ulim/1 -> 2nd order fdbk for ulim/1
  defl_cmd/1 -> 2nd order fdbk for cmd/1
  defl_llim/1 -> 2nd order fdbk for llim/1
  [defl] -> 2nd order fdbk for ulim/2
  [defl] -> 2nd order fdbk for cmd/2
  [defl] -> 2nd order fdbk for llim/2
  [defld] -> 2nd order fdbk for ulim/3
  [defld] -> 1st order fdbk for urlim/2
  [defld] -> 2nd order fdbk for cmd/3
  [defld] -> 1st order fdbk for lrlim/2
  [defld] -> 2nd order fdbk for llim/3
  1st order fdbk for urlim/1 -> MinMax/1
  defl_urlim/1 -> 1st order fdbk for urlim/1
  defl_lrlim/1 -> 1st order fdbk for lrlim/1
  1st order fdbk for lrlim/1 -> MinMax1/2
  Constant1/1 -> 2nd order fdbk for ulim/5
  Constant2/1 -> 2nd order fdbk for llim/5
  zeta/1 -> 2nd order fdbk for cmd/5
  w/1 -> 2nd order fdbk for llim/4, 1st order fdbk for lrlim/3, 2nd order fdbk for cmd/4, 2nd order fdbk for ulim/4, 1st order fdbk for urlim/3
  MinMax2/1 -> MinMax3/1
  MinMax3/1 -> defldd/1
  2nd order fdbk for llim/1 -> MinMax3/2
  2nd order fdbk for ulim/1 -> MinMax2/1
  MinMax1/1 -> MinMax2/2
  2nd order fdbk for cmd/1 -> MinMax/2
  defld/1 -> [defld]
  defl/1 -> [defl]

== system model_lib/variable limit servo model ==
  note: VARIABLE LIMIT SERVO MODEL
  act_bus : Inport
  2*Z*W : Gain  Orientation=left  Gain=2*SERVO.z.*SERVO.w  SaturateOnIntegerOverflow=on
  Bus Selector1 : BusSelector  OutputSignals=effector_limits.u_ulim,effector_limits.u_llim,u_cmd
  Enforce lower limit : MinMax  Function=max  Inputs=2  OutScaling=2^-10  ZeroCross=off
  Enforce upper limit : MinMax  Inputs=2  OutScaling=2^-10  ZeroCross=off
  Rate Limiter : RateLimiter  RisingSlewLimit=SERVO.urlim  FallingSlewLimit=SERVO.lrlim  SampleTimeMode=inherited  InitialCondition=SERVO.x0
  Sum : Sum  Inputs=|+-  SaturateOnIntegerOverflow=on  InputSameDT=on
  Sum1 : Sum  Inputs=|++  SaturateOnIntegerOverflow=on  InputSameDT=on
  Sum2 : Sum  Orientation=left  Inputs=-+|  SaturateOnIntegerOverflow=on  InputSameDT=on
  Sum3 : Sum  Inputs=|+-  SaturateOnIntegerOverflow=on  InputSameDT=on
  W^2 : Gain  Gain=SERVO.w.^2  SaturateOnIntegerOverflow=on
  anti-windup gain : Gain  Orientation=left  Gain=SERVO.pos_Kaw
  pos integrator : Integrator  InitialCondition=SERVO.x0
  rate integrator : Integrator  LimitOutput=on  UpperSaturationLimit=SERVO.urlim  LowerSaturationLimit=SERVO.lrlim
  u_pos : Outport
  wires:
  Enforce upper limit/1 -> Rate Limiter/1
  Enforce lower limit/1 -> Enforce upper limit/2
  pos integrator/1 -> Sum2/1, Enforce lower limit/2
  Sum2/1 -> anti-windup gain/1
  anti-windup gain/1 -> Sum1/2
  Sum1/1 -> pos integrator/1
  rate integrator/1 -> Sum1/1, 2*Z*W/1
  Sum/1 -> W^2/1
  Sum3/1 -> rate integrator/1
  W^2/1 -> Sum3/1
  2*Z*W/1 -> Sum3/2
  Rate Limiter/1 -> u_pos/1, Sum2/2, Sum/2
  act_bus/1 -> Bus Selector1/1
  Bus Selector1/3 -> Sum/1  "<u_cmd>"
  Bus Selector1/2 -> Enforce lower limit/1  "<u_llim>"
  Bus Selector1/1 -> Enforce upper limit/1  "<u_ulim>"

== system model_lib/variable rate limit discrete servo model ==
  note: VARIABLE RATE LIMIT DISCRETE SERVO MODEL
  act_bus : Inport
  Bus Selector1 : BusSelector  OutputSignals=u_cmd,effector_limits.u_ulim,effector_limits.u_llim,effector_limits.u_urlim,effector_limits.u_lrlim
  Constant : Constant  Value=SERVO.z
  Constant1 : Constant  Value=SERVO.w
  defl integrator : DiscreteIntegrator  InitialCondition=SERVO.x0  SampleTime=-1  ICPrevOutput=DiscIntNeverNeededParam  ICPrevScaledInput=DiscIntNeverNeededParam
  defld integrator : DiscreteIntegrator  SampleTime=-1  ICPrevOutput=DiscIntNeverNeededParam  ICPrevScaledInput=DiscIntNeverNeededParam
  variable limit servo core : model_lib/variable limit servo core
  u_pos : Outport
  wires:
  Constant/1 -> variable limit servo core/7
  Constant1/1 -> variable limit servo core/6
  Bus Selector1/5 -> variable limit servo core/5  "<u_lrlim>"
  Bus Selector1/4 -> variable limit servo core/4  "<u_urlim>"
  Bus Selector1/3 -> variable limit servo core/3  "<u_llim>"
  Bus Selector1/2 -> variable limit servo core/2  "<u_ulim>"
  Bus Selector1/1 -> variable limit servo core/1  "<u_cmd>"
  defld integrator/1 -> variable limit servo core/9, defl integrator/1
  variable limit servo core/1 -> defld integrator/1
  defl integrator/1 -> u_pos/1, variable limit servo core/8
  act_bus/1 -> Bus Selector1/1

== system model_lib/variable rate limit servo model ==
  note: VARIABLE RATE LIMIT SERVO MODEL
  act_bus : Inport
  Bus Selector1 : BusSelector  OutputSignals=u_cmd,effector_limits.u_ulim,effector_limits.u_llim,effector_limits.u_urlim,effector_limits.u_lrlim
  Constant : Constant  Value=SERVO.z
  Constant1 : Constant  Value=SERVO.w
  defl integrator : Integrator  InitialCondition=SERVO.x0
  defld integrator : Integrator
  variable limit servo core : model_lib/variable limit servo core
  u_pos : Outport
  wires:
  act_bus/1 -> Bus Selector1/1
  defl integrator/1 -> variable limit servo core/8, u_pos/1
  variable limit servo core/1 -> defld integrator/1
  defld integrator/1 -> defl integrator/1, variable limit servo core/9
  Bus Selector1/1 -> variable limit servo core/1  "<u_cmd>"
  Bus Selector1/2 -> variable limit servo core/2  "<u_ulim>"
  Bus Selector1/3 -> variable limit servo core/3  "<u_llim>"
  Bus Selector1/4 -> variable limit servo core/4  "<u_urlim>"
  Bus Selector1/5 -> variable limit servo core/5  "<u_lrlim>"
  Constant1/1 -> variable limit servo core/6
  Constant/1 -> variable limit servo core/7

== system model_lib/Sensor Errors/Sensor A/D Quantization ==
  note: Sensor Analog-to-Digital Quantization
  note: select quantization model 1 or 2
      | 1=> Perfect
      |  2=> Quantizize
  y : Inport
  " Quantization" : Quantizer  QuantizationInterval=ADQUANT.interval  SampleTime=dtsim
  Constant : Constant  Value=ADQUANT.model
  Multiport Switch : MultiPortSwitch  Inputs=2  SaturateOnIntegerOverflow=on  InputSameDT=on
  yQ : Outport
  wires:
  Multiport Switch/1 -> yQ/1
  y/1 -> Multiport Switch/2, " Quantization"/1
  Constant/1 -> Multiport Switch/1
  " Quantization"/1 -> Multiport Switch/3

== system model_lib/Sensor Errors/Sensor Errors ==
  note: Sensor Errors
  note: select servo model 1 or 2
      | 1=> Perfect
      |  2=>Sensor Model
  y : Inport
  " Constant" : Constant  Value=SENS.model
  Multiport Switch : MultiPortSwitch  Inputs=2  SaturateOnIntegerOverflow=on  InputSameDT=on
  "Sensor Model " : Subsystem
  normalize quaternions : Subsystem
  ys : Outport
  wires:
  y/1 -> Multiport Switch/2, "Sensor Model "/1(y)
  Multiport Switch/1 -> ys/1
  " Constant"/1 -> Multiport Switch/1
  "Sensor Model "/1(y_sens) -> normalize quaternions/1(y_sens_in)
  normalize quaternions/1(y_sens_out) -> Multiport Switch/3

== system model_lib/get atmos_env/air density ==
  h : Inport
  Constant1 : Constant  Value=rho_sl
  Constant2 : Constant  Value=alt_ht
  Product : Product  RndMeth=Zero
  Sum : Sum  Inputs=|-+
  stratosphere : Subsystem
  troposphere : Subsystem
  u2>=0 : Switch
  rho : Outport
  wires:
  h/1 -> troposphere/1(h), stratosphere/1(h), Sum/1
  troposphere/1(sig) -> u2>=0/1
  stratosphere/1(sig) -> u2>=0/3
  Constant2/1 -> Sum/2
  Sum/1 -> u2>=0/2
  Constant1/1 -> Product/2
  u2>=0/1 -> Product/1
  Product/1 -> rho/1

== system model_lib/get atmos_env/air temp ==
  h : Inport
  Constant2 : Constant  Value=alt_ht
  Sum : Sum  Inputs=|-+
  stratosphere : Subsystem
  troposphere : Subsystem
  u2>=0 : Switch
  T : Outport
  wires:
  u2>=0/1 -> T/1
  Sum/1 -> u2>=0/2
  Constant2/1 -> Sum/2
  stratosphere/1(T) -> u2>=0/3
  troposphere/1(T) -> u2>=0/1
  h/1 -> troposphere/1(h), Sum/1

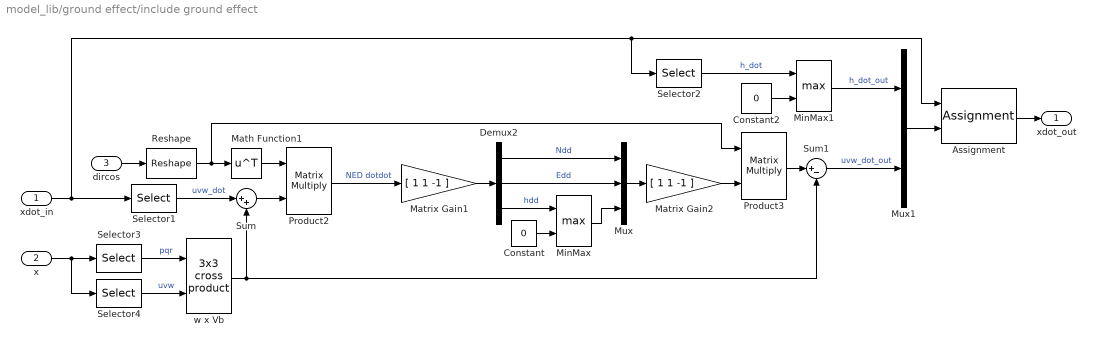
== system model_lib/ground effect/include ground effect ==
  xdot_in : Inport
  x : Inport  Port=2
  dircos : Inport  Port=3
  Assignment : Assignment  Elements=[MACH.NEh_idx(3) MACH.uvw_idx]  OutputInitialize=Initialize using input (U1)
  Constant : Constant  Value=0
  Constant2 : Constant  Value=0
  Demux2 : Demux  Outputs=3
  Math Function1 : Math  Operator=transpose  SaturateOnIntegerOverflow=on
  Matrix Gain1 : Gain  Gain=[ 1 1 -1 ]  SaturateOnIntegerOverflow=on
  Matrix Gain2 : Gain  Gain=[ 1 1 -1 ]  SaturateOnIntegerOverflow=on
  MinMax : MinMax  Function=max  Inputs=2  SaturateOnIntegerOverflow=on  InputSameDT=on
  MinMax1 : MinMax  Function=max  Inputs=2  SaturateOnIntegerOverflow=on  InputSameDT=on
  Mux : Mux  Inputs=3
  Mux1 : Mux  Inputs=2
  Product2 : Product  Multiplication=Matrix(*)  SaturateOnIntegerOverflow=on  InputSameDT=on
  Product3 : Product  Multiplication=Matrix(*)  SaturateOnIntegerOverflow=on  InputSameDT=on
  Reshape : simulink/Math Operations/Reshape  OutputDimensionality=Customize  OutputDimensions=[3,3]
  Selector1 : Selector  Elements=MACH.uvw_idx  InputPortWidth=num_x
  Selector2 : Selector  Elements=MACH.NEh_idx(3)  InputPortWidth=num_x
  Selector3 : Selector  Elements=MACH.pqr_idx  InputPortWidth=num_x
  Selector4 : Selector  Elements=MACH.uvw_idx  InputPortWidth=num_x
  Sum : Sum  Inputs=|++  SaturateOnIntegerOverflow=on
  Sum1 : Sum  Inputs=|+-  SaturateOnIntegerOverflow=on
  w x Vb : aerospace/Axes Transformations/3x3 cross product
  xdot_out : Outport
  wires:
  Product2/1 -> Matrix Gain1/1  "NED dotdot"
  Matrix Gain2/1 -> Product3/2
  Reshape/1 -> Math Function1/1, Product3/1
  xdot_in/1 -> Selector1/1, Selector2/1, Assignment/1
  Matrix Gain1/1 -> Demux2/1
  Mux/1 -> Matrix Gain2/1
  Math Function1/1 -> Product2/1
  Demux2/1 -> Mux/1  "Ndd"
  Demux2/2 -> Mux/2  "Edd"
  Constant/1 -> MinMax/2
  Demux2/3 -> MinMax/1  "hdd"
  MinMax/1 -> Mux/3
  dircos/1 -> Reshape/1
  Constant2/1 -> MinMax1/2
  MinMax1/1 -> Mux1/1  "h_dot_out"
  Selector2/1 -> MinMax1/1  "h_dot"
  x/1 -> Selector3/1, Selector4/1
  Selector3/1 -> w x Vb/1  "pqr"
  Selector4/1 -> w x Vb/2  "uvw"
  Selector1/1 -> Sum/1  "uvw_dot"
  Sum/1 -> Product2/2
  w x Vb/1 -> Sum/2, Sum1/2
  Product3/1 -> Sum1/1
  Sum1/1 -> Mux1/2  "uvw_dot_out"
  Mux1/1 -> Assignment/2
  Assignment/1 -> xdot_out/1

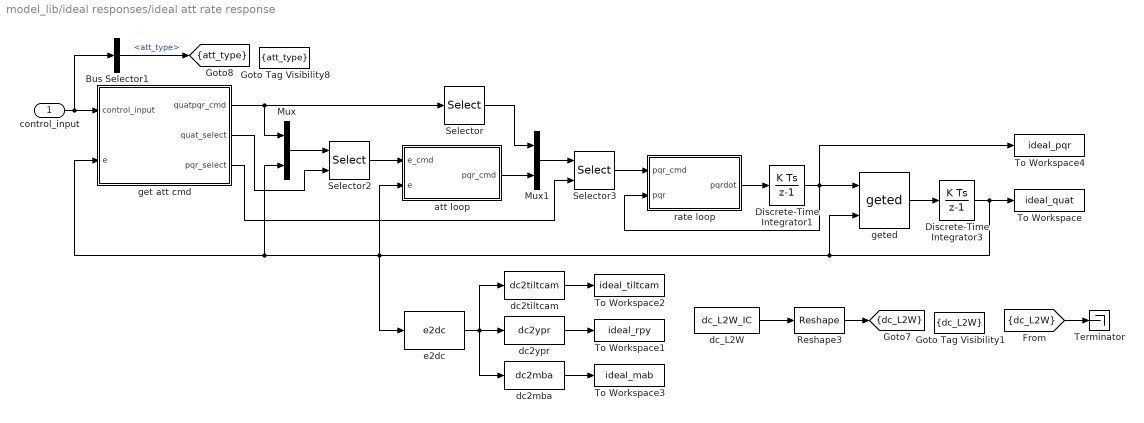
== system model_lib/ideal responses/ideal att rate response ==
  control_input : Inport
  Bus Selector1 : BusSelector  OutputSignals=mode_sw.att_type
  Discrete-Time Integrator1 : DiscreteIntegrator  InitialCondition=MACH_pqr_IC  SampleTime=-1  ICPrevOutput=DiscIntNeverNeededParam  ICPrevScaledInput=DiscIntNeverNeededParam
  Discrete-Time Integrator3 : DiscreteIntegrator  InitialCondition=MACH_quat_IC  SampleTime=-1  ICPrevOutput=DiscIntNeverNeededParam  ICPrevScaledInput=DiscIntNeverNeededParam
  Goto Tag Visibility1 : GotoTagVisibility  GotoTag=dc_L2W
  Goto Tag Visibility8 : GotoTagVisibility  GotoTag=att_type
  Mux : Mux  Inputs=2
  Mux1 : Mux  Inputs=2
  Reshape3 : simulink/Math Operations/Reshape  OutputDimensionality=1-D array  OutputDimensions=[3 3]
  Selector : Selector  Elements=[1 2 3]  InputPortWidth=4
  Selector2 : Selector  ElementSrc=External  Elements=[4 5 3]  InputPortWidth=8
  Selector3 : Selector  ElementSrc=External  Elements=[1 2 6]  InputPortWidth=6
  Terminator : Terminator
  To Workspace : ToWorkspace  VariableName=ideal_quat  SampleTime=MACH.dt  SaveFormat=Array
  To Workspace1 : ToWorkspace  VariableName=ideal_rpy  SampleTime=MACH.dt  SaveFormat=Array
  To Workspace2 : ToWorkspace  VariableName=ideal_tiltcam  SampleTime=MACH.dt  SaveFormat=Array
  To Workspace3 : ToWorkspace  VariableName=ideal_mab  SampleTime=MACH.dt  SaveFormat=Array
  To Workspace4 : ToWorkspace  VariableName=ideal_pqr  SampleTime=MACH.dt  SaveFormat=Array
  att loop : Subsystem
  dc2mba : utility_lib/dc2mba
  dc2tiltcam : utility_lib/dc2tiltcam
  dc2ypr : utility_lib/dc2ypr
  dc_L2W : Constant  Value=dc_L2W_IC
  e2dc : utility_lib/e2dc
  get att cmd : Subsystem
  geted : utility_lib/geted
  rate loop : Subsystem
  tag scope: att_type=scoped, dc_L2W=scoped
  wires:
  Discrete-Time Integrator3/1 -> To Workspace/1, geted/2, e2dc/1, att loop/2(e), Mux/2, get att cmd/2(e)
  geted/1 -> Discrete-Time Integrator3/1
  get att cmd/1(quatpqr_cmd) -> Selector/1, Mux/1
  rate loop/1(pqrdot) -> Discrete-Time Integrator1/1
  dc_L2W/1 -> Reshape3/1
  Reshape3/1 -> [dc_L2W]
  [dc_L2W] -> Terminator/1
  e2dc/1 -> dc2ypr/1, dc2mba/1, dc2tiltcam/1
  dc2tiltcam/1 -> To Workspace2/1
  dc2ypr/1 -> To Workspace1/1
  dc2mba/1 -> To Workspace3/1
  control_input/1 -> get att cmd/1(control_input), Bus Selector1/1
  Discrete-Time Integrator1/1 -> geted/1, rate loop/2(pqr), To Workspace4/1
  Selector3/1 -> rate loop/1(pqr_cmd)
  Mux1/1 -> Selector3/1
  att loop/1(pqr_cmd) -> Mux1/2
  Selector/1 -> Mux1/1
  get att cmd/3(pqr_select) -> Selector3/2
  Selector2/1 -> att loop/1(e_cmd)
  Mux/1 -> Selector2/1
  get att cmd/2(quat_select) -> Selector2/2
  Bus Selector1/1 -> [att_type]  "<att_type>"
